simulink model "Group1.control_submission"  (R2024a)
settings: Solver=VariableStepAuto  StartTime=0.0  StopTime=10.0  RelTol=1e-3
undefined symbols (not defined in the file or in its folder): Ts
settings Model: Creator=Riley  LastModifiedBy=Riley

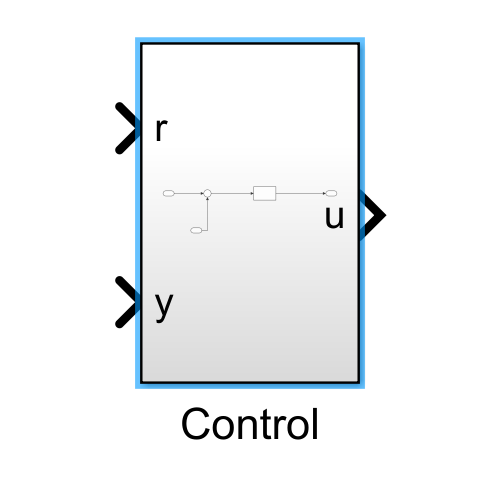
[thumbnail: Simulink's stored preview of the top-level diagram]
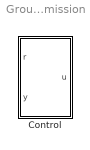
== system Group1.control_submission ==
  Control : Subsystem

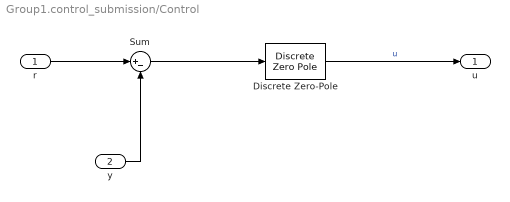
== system Group1.control_submission/Control ==
  r : Inport
  y : Inport  Port=2
  Discrete Zero-Pole : DiscreteZeroPole  Zeros=[0.98683+0.16207i;0.98683-0.16207i]  Poles=[0.83754+2.4407e-07i, 0.83754-2.4407e-07i]  Gain=0.30424  SampleTime=Ts
  Sum : Sum  Inputs=|+-
  u : Outport
  wires:
  Sum/1 -> Discrete Zero-Pole/1
  r/1 -> Sum/1
  Discrete Zero-Pole/1 -> u/1  "u"
  y/1 -> Sum/2
